simulink model "directVectorControl"  (R2023a)
settings: Solver=VariableStepAuto  StartTime=0.0  StopTime=3  MaxStep=.00001  RelTol=.00001
values from neighbouring files (symbols this model uses):
  B = .005752    (= 0.005752)    [parameters.m]
  Fs = 5000    [parameters.m]
  I_rated = P_rated/(sqrt(3)*VLL_rms*.9*.9)    [parameters.m]
  Id_rated = lambda_r_rated/Lm    (= 3.46097201767)    [parameters.m]
  J = .02    (= 0.02)    [parameters.m]
  lambda_r_rated = 0.705    [parameters.m]
  Llr = .005974    (= 0.005974)    [parameters.m]
  Lls = .005974    (= 0.005974)    [parameters.m]
  Lm = .2037    (= 0.2037)    [parameters.m]
  Lr = Lm+Llr    (= 0.209674)    [parameters.m]
  Ls = Lm+Lls    (= 0.209674)    [parameters.m]
  P = 4    [parameters.m]
  Rs = 1.115    [parameters.m]
  sigma = 1-((Lm)^2)/(Lr*Ls)    (= 0.0561719130296)    [parameters.m]
  Tr = Lr/Rr    (= 0.193604801477)    [parameters.m]
  Vdc = 650    [parameters.m]
libraries: slpidlib x8, spsMosfetLib x6, spsabctoAlphaBetaZeroLib x4, spsCurrentMeasurementLib x2, simulink x2, SignalEditorBlockLib x2, spsAsynchronousMachineSIUnitsLib x1, spsDCVoltageSourceLib x1, spspowerguiLib x1
(part 2 of 2)

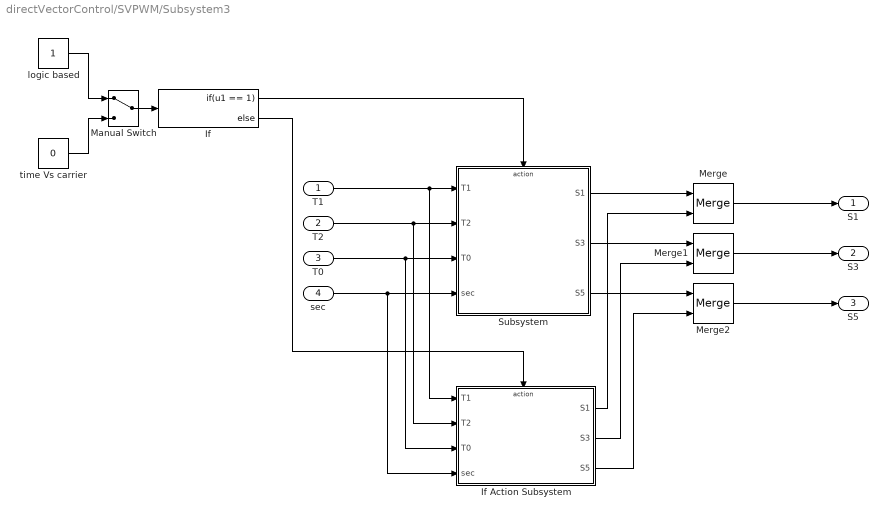
== system directVectorControl/SVPWM/Subsystem3 ==
  T1 : Inport
  T2 : Inport  Port=2
  T0 : Inport  Port=3
  sec : Inport  Port=4
  If : If  IfExpression=u1 == 1
  If Action Subsystem : Subsystem  TreatAsAtomicUnit=on
  Manual Switch : ManualSwitch
  Merge : Merge
  Merge1 : Merge
  Merge2 : Merge
  Subsystem : Subsystem
  logic based : Constant
  time Vs carrier : Constant  Value=0
  S1 : Outport
  S3 : Outport  Port=2
  S5 : Outport  Port=3
  wires:
  T1/1 -> If Action Subsystem/1(T1), Subsystem/1(T1)
  T2/1 -> If Action Subsystem/2(T2), Subsystem/2(T2)
  T0/1 -> If Action Subsystem/3(T0), Subsystem/3(T0)
  sec/1 -> If Action Subsystem/4(sec), Subsystem/4(sec)
  Merge/1 -> S1/1
  Merge1/1 -> S3/1
  Merge2/1 -> S5/1
  Manual Switch/1 -> If/1
  logic based/1 -> Manual Switch/1
  time Vs carrier/1 -> Manual Switch/2
  If/1 -> Subsystem/Action
  If/2 -> If Action Subsystem/Action
  Subsystem/1(S1) -> Merge/1
  Subsystem/2(S3) -> Merge1/1
  Subsystem/3(S5) -> Merge2/1
  If Action Subsystem/1(S1) -> Merge/2
  If Action Subsystem/2(S3) -> Merge1/2
  If Action Subsystem/3(S5) -> Merge2/2

== system directVectorControl/Subsystem/Constant Power region ==
  Action Port : ActionPort  ActionPortLabel=else
  Rated Flux : Constant  Value=lambda_r_rated
  λdr : Outport
  Iqs_max : Outport  Port=2
  wires:
  Rated Flux/1 -> λdr/1  "λdr*"
  ? -> Iqs_max/1

== system directVectorControl/Subsystem/Constant Torque region ==
  Action Port : ActionPort  ActionPortLabel=if(u1 < Wr_base)
  Constant : Constant  Value=I_rated
  Gain : Gain  Gain=1/Lm
  Rated Flux : Constant  Value=lambda_r_rated
  Sqrt : Sqrt
  Square : Math  Operator=square
  Square1 : Math  Operator=square
  Subtract : Sum  Inputs=-+
  λdr : Outport
  Iqs_max : Outport  Port=2
  wires:
  Rated Flux/1 -> Gain/1, λdr/1  "λdr*"
  Gain/1 -> Square/1  "Idr"
  Square/1 -> Subtract/1
  Constant/1 -> Square1/1
  Square1/1 -> Subtract/2
  Sqrt/1 -> Iqs_max/1
  Subtract/1 -> Sqrt/1

== system directVectorControl/SVPWM/Subsystem2/Subsystem ==
  θ : Inport
  sec : Inport  Port=2
  Constant : Constant
  Constant1 : Constant  Value=pi/3
  Product : Product
  Subtract : Sum  Inputs=+-
  Subtract1 : Sum  Inputs=+-
  θ` : Outport
  wires:
  θ/1 -> Subtract/1
  sec/1 -> Subtract1/1
  Constant/1 -> Subtract1/2
  Subtract1/1 -> Product/1
  Subtract/1 -> θ`/1
  Constant1/1 -> Product/2
  Product/1 -> Subtract/2

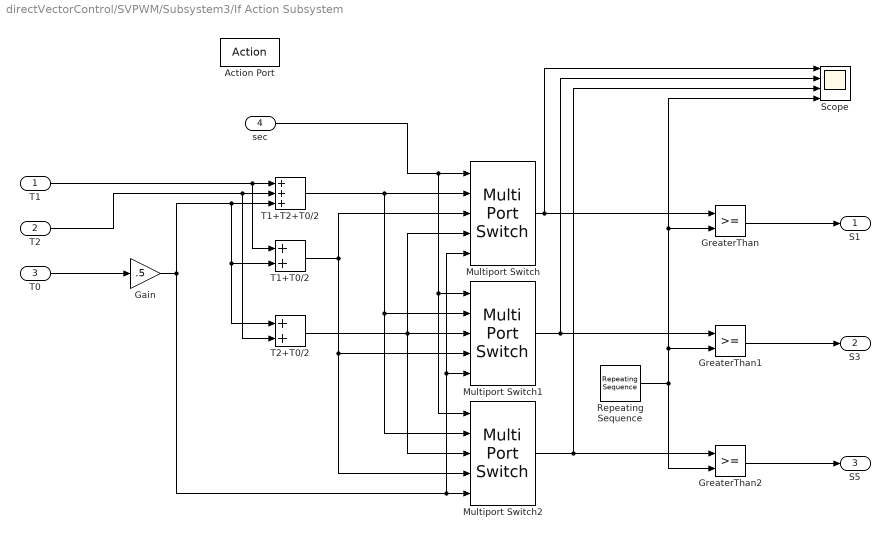
== system directVectorControl/SVPWM/Subsystem3/If Action Subsystem ==
  T1 : Inport
  T2 : Inport  Port=2
  T0 : Inport  Port=3
  sec : Inport  Port=4
  Action Port : ActionPort  ActionPortLabel=else
  Gain : Gain  Gain=.5
  GreaterThan : RelationalOperator  OutDataTypeStr=boolean  RndMeth=Simplest  InputSameDT=off
  GreaterThan1 : RelationalOperator  OutDataTypeStr=boolean  RndMeth=Simplest  InputSameDT=off
  GreaterThan2 : RelationalOperator  OutDataTypeStr=boolean  RndMeth=Simplest  InputSameDT=off
  Multiport Switch : MultiPortSwitch  DataPortOrder=Specify indices  DataPortIndices={[1,6],2,5,[3,4]}  SaturateOnIntegerOverflow=off  InputSameDT=off
  Multiport Switch1 : MultiPortSwitch  DataPortOrder=Specify indices  DataPortIndices={[2,3],1,4,[5,6]}  SaturateOnIntegerOverflow=off  InputSameDT=off
  Multiport Switch2 : MultiPortSwitch  DataPortOrder=Specify indices  DataPortIndices={[4,5],3,6,[1,2]}  SaturateOnIntegerOverflow=off  InputSameDT=off
  Repeating Sequence : simulink/Sources/Repeating Sequence  rep_seq_t=[0 1 2]/(Fs)  rep_seq_y=[0 1 0]/(Fs)
  Scope : Scope  NumInputPorts=4
  T1+T0/2 : Sum
  T1+T2+T0/2 : Sum  Inputs=+++
  T2+T0/2 : Sum
  S1 : Outport
  S3 : Outport  Port=2
  S5 : Outport  Port=3
  wires:
  T0/1 -> Gain/1
  T1/1 -> T1+T0/2/1, T1+T2+T0/2/1
  T2/1 -> T2+T0/2/2, T1+T2+T0/2/2
  Gain/1 -> T1+T2+T0/2/3, T2+T0/2/1, T1+T0/2/2, Multiport Switch1/5, Multiport Switch/5, Multiport Switch2/5
  sec/1 -> Multiport Switch1/1, Multiport Switch2/1, Multiport Switch/1
  T1+T0/2/1 -> Multiport Switch/3, Multiport Switch2/4, Multiport Switch1/4
  T2+T0/2/1 -> Multiport Switch2/3, Multiport Switch1/3, Multiport Switch/4
  T1+T2+T0/2/1 -> Multiport Switch/2, Multiport Switch2/2, Multiport Switch1/2
  Multiport Switch/1 -> GreaterThan/1, Scope/1
  Multiport Switch2/1 -> Scope/3, GreaterThan2/1
  Multiport Switch1/1 -> GreaterThan1/1, Scope/2
  Repeating Sequence/1 -> GreaterThan2/2, Scope/4, GreaterThan/2, GreaterThan1/2
  GreaterThan/1 -> S1/1
  GreaterThan1/1 -> S3/1
  GreaterThan2/1 -> S5/1

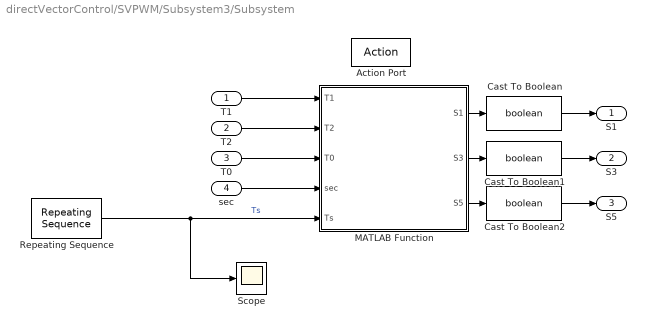
== system directVectorControl/SVPWM/Subsystem3/Subsystem ==
  T1 : Inport
  T2 : Inport  Port=2
  T0 : Inport  Port=3
  sec : Inport  Port=4
  Action Port : ActionPort  ActionPortLabel=if(u1 == 1)
  Cast To Boolean : DataTypeConversion  OutDataTypeStr=boolean  SaturateOnIntegerOverflow=off  RndMeth=Floor
  Cast To Boolean1 : DataTypeConversion  OutDataTypeStr=boolean  SaturateOnIntegerOverflow=off  RndMeth=Floor
  Cast To Boolean2 : DataTypeConversion  OutDataTypeStr=boolean  SaturateOnIntegerOverflow=off  RndMeth=Floor
  MATLAB Function : MATLAB Function  TreatAsAtomicUnit=on
  Repeating Sequence : simulink/Sources/Repeating Sequence  rep_seq_t=[0 1/Fs]  rep_seq_y=[0 1/Fs]
  Scope : Scope
  S1 : Outport
  S3 : Outport  Port=2
  S5 : Outport  Port=3
  wires:
  Repeating Sequence/1 -> MATLAB Function/5(Ts), Scope/1  "Ts"
  T2/1 -> MATLAB Function/2(T2)
  sec/1 -> MATLAB Function/4(sec)
  T1/1 -> MATLAB Function/1(T1)
  MATLAB Function/2(S3) -> Cast To Boolean1/1
  T0/1 -> MATLAB Function/3(T0)
  MATLAB Function/3(S5) -> Cast To Boolean2/1
  MATLAB Function/1(S1) -> Cast To Boolean/1
  Cast To Boolean/1 -> S1/1
  Cast To Boolean1/1 -> S3/1
  Cast To Boolean2/1 -> S5/1

== matlab function directVectorControl/SVPWM/Subsystem3/Subsystem/MATLAB Function ==
  data: T1 input; S1 output; T2 input; T0 input; sec input; Ts input; S3 output; S5 output
function [S1,S3, S5] = fcn(T1, T2, T0, sec, Ts)
%|--T0/4--||----T1/2----||----T2/2----||----T7/2----||----T2/2----||----T2/2----||--T0/4--|
%         reg1           reg2          reg3          reg4          reg5         reg6      Ts       
S1=0;
S3=0;
S5=0;
if (sec == 2) || (sec==4) || (sec==6)
temp=T1;
T1=T2;
T2=temp;
end
reg1=T0/4;
reg2=reg1+(T1/2);
reg3=reg2+(T2/2);
reg4=reg3+(T0/2);
reg5=reg4+(T2/2);
reg6=reg5+(T1/2);

switch sec

       %----------------------First sector----------------------%
   case 1
        if(Ts>reg1) && (Ts<=reg6)
            S1=1;
        else
            S1=0;
        end

        if (Ts > reg2) && (Ts <= reg5)
            S3=1;
        else
            S3=0;
        end
        if (Ts > reg3) && (Ts <= reg4)
            S5=1;
        else
            S5=0;
        end

        %----------------------Second sector----------------------%
    case 2
        if (Ts > reg2) && (Ts <= reg5)
            S1=1;
        else
            S1=0;
        end
        if(Ts>reg1) && (Ts<=reg6)
            S3=1;
        else
            S3=0;
        end
        if (Ts > reg3) && (Ts <= reg4)
            S5=1;
        else
            S5=0;
        end

        %----------------------third sector----------------------%
    case 3
        if (Ts > reg3) && (Ts <= reg4)
            S1=1;
        else
            S1=0;
        end
        if(Ts>reg1) && (Ts<=reg6)
            S3=1;
        else
            S3=0;
        end
        if (Ts > reg2) && (Ts <= reg5)
            S5=1;
        else
            S5=0;
        end

        %----------------------4th sector----------------------%
   case 4
        if (Ts > reg3) && (Ts <= reg4)
            S1=1;
        else
            S1=0;
        end
        if (Ts > reg2) && (Ts <= reg5)
            S3=1;
        else
            S3=0;
        end
        if(Ts>reg1) && (Ts<=reg6)
            S5=1;
        else
            S5=0;
        end

        %----------------------5th sector----------------------%
    case 5
        if (Ts > reg2) && (Ts <= reg5)
            S1=1;
        else
            S1=0;
        end
        if (Ts > reg3) && (Ts <= reg4)
            S3=1;
        else
            S3=0;
        end
        if(Ts>reg1) && (Ts<=reg6)
            S5=1;
        else
            S5=0;
        end
        
        %----------------------6th sector----------------------%
    case 6
        if(Ts>reg1) && (Ts<=reg6)
            S1=1;
        else
            S1=0;
        end
        if (Ts > reg3) && (Ts <= reg4)
            S3=1;
        else
            S3=0;
        end
        if (Ts > reg2) && (Ts <= reg5)
            S5=1;
        else
            S5=0;
        end
end
end

== matlab function directVectorControl/SVPWM/sector detection ==
  data: theta input; sec output
function sec = fcn(theta)
sec=0;
if ((theta >= 0) && (theta <=60))
    sec =1;
elseif (((theta > 60) && (theta <=120)))
    sec =2;
elseif (((theta > 120) && (theta <= 180)))
    sec =3;
elseif (((theta > 180) && (theta <= 240)))
    sec =4;
elseif (((theta > 240) && (theta <= 300)))
    sec =5;
elseif (((theta > 300) && (theta <= 360)))
    sec =6;
end
end
